simulink model "freq_detection_algorithm"  (R2021a)
settings: Solver=VariableStepAuto  StartTime=0.0  StopTime=10.0  RelTol=1e-3
Description:
  | Model is intend to simulate calculations for a flowmeter.
settings Model: Creator=Ayush  LastModifiedBy=Ayush

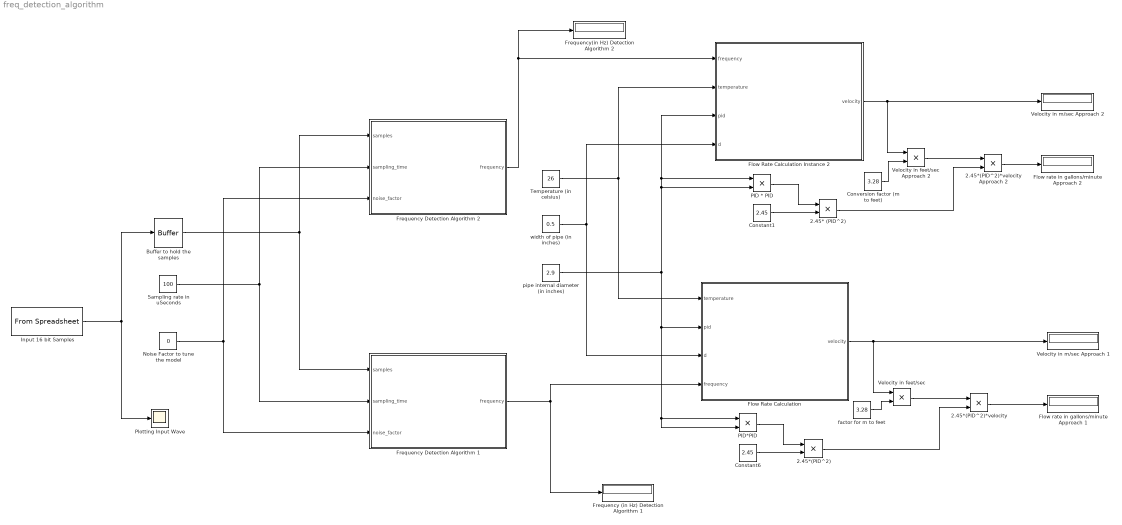
== system freq_detection_algorithm ==
  2.45* (PID^2) : Product
  2.45*(PID^2) : Product
  2.45*(PID^2)*velocity : Product
  2.45*(PID^2)*velocity Approach 2 : Product
  Buffer to hold the samples : Buffer  N=1000  OutputFrames=off
  Constant1 : Constant  Value=2.45  SampleTime=0.0005
  Constant6 : Constant  Value=2.45  SampleTime=0.0005
  Conversion factor (m to feet) : Constant  Value=3.28  SampleTime=0.0005
  Flow Rate Calculation : MATLAB Function  TreatAsAtomicUnit=on
  Flow Rate Calculation Instance 2 : MATLAB Function  TreatAsAtomicUnit=on
  Flow rate in gallons/minute Approach 1 : Display
  Flow rate in gallons/minute Approach 2 : Display
  Frequency (in Hz) Detection Algorithm 1 : Display
  Frequency Detection Algorithm 1 : MATLAB Function  TreatAsAtomicUnit=on
  Frequency Detection Algorithm 2 : MATLAB Function  TreatAsAtomicUnit=on
  Frequency(in Hz) Detection Algorithm 2 : Display
  Input 16 bit Samples : FromSpreadsheet  FileName=ECEN5803Data17_1.csv  SheetName=ECEN5803Data17_1  OutDataTypeStr=double  TreatFirstColumnAs=Data  SampleTime=0.0001
  Noise Factor to tune the model : Constant  Value=0  SampleTime=0.00001
  PID * PID : Product
  PID*PID : Product
  Plotting Input Wave : Scope
  Sampling rate in uSeconds : Constant  Value=100  SampleTime=100
  Temperature (in celsius) : Constant  Value=26  SampleTime=0.0005
  Velocity in feet/sec : Product
  Velocity in feet/sec Approach 2 : Product
  Velocity in m/sec Approach 1 : Display
  Velocity in m/sec Approach 2 : Display
  factor for m to feet : Constant  Value=3.28  SampleTime=0.0005
  pipe internal diameter (in inches) : Constant  Value=2.9  SampleTime=100
  width of pipe (in inches) : Constant  Value=0.5  SampleTime=100
  wires:
  Buffer to hold the samples/1 -> Frequency Detection Algorithm 2/1(samples), Frequency Detection Algorithm 1/1(samples)
  Sampling rate in uSeconds/1 -> Frequency Detection Algorithm 2/2(sampling_time), Frequency Detection Algorithm 1/2(sampling_time)
  Noise Factor to tune the model/1 -> Frequency Detection Algorithm 2/3(noise_factor), Frequency Detection Algorithm 1/3(noise_factor)
  Frequency Detection Algorithm 1/1(frequency) -> Flow Rate Calculation/4(frequency), Frequency (in Hz) Detection Algorithm 1/1
  Input 16 bit Samples/1 -> Buffer to hold the samples/1, Plotting Input Wave/1
  Flow Rate Calculation/1(velocity) -> Velocity in feet/sec/1, Velocity in m/sec Approach 1/1
  factor for m to feet/1 -> Velocity in feet/sec/2
  Velocity in feet/sec/1 -> 2.45*(PID^2)*velocity/1
  2.45*(PID^2)*velocity/1 -> Flow rate in gallons/minute Approach 1/1
  PID*PID/1 -> 2.45*(PID^2)/1
  Constant6/1 -> 2.45*(PID^2)/2
  2.45*(PID^2)/1 -> 2.45*(PID^2)*velocity/2
  Frequency Detection Algorithm 2/1(frequency) -> Frequency(in Hz) Detection Algorithm 2/1, Flow Rate Calculation Instance 2/1(frequency)
  2.45* (PID^2)/1 -> 2.45*(PID^2)*velocity Approach 2/2
  Constant1/1 -> 2.45* (PID^2)/2
  2.45*(PID^2)*velocity Approach 2/1 -> Flow rate in gallons/minute Approach 2/1
  Velocity in feet/sec Approach 2/1 -> 2.45*(PID^2)*velocity Approach 2/1
  Flow Rate Calculation Instance 2/1(velocity) -> Velocity in feet/sec Approach 2/1, Velocity in m/sec Approach 2/1
  PID * PID/1 -> 2.45* (PID^2)/1
  Temperature (in celsius)/1 -> Flow Rate Calculation/1(temperature), Flow Rate Calculation Instance 2/2(temperature)
  width of pipe (in inches)/1 -> Flow Rate Calculation Instance 2/4(d), Flow Rate Calculation/3(d)
  pipe internal diameter (in inches)/1 -> Flow Rate Calculation/2(pid), PID*PID/1, PID*PID/2, PID * PID/2, PID * PID/1, Flow Rate Calculation Instance 2/3(pid)
  Conversion factor (m to feet)/1 -> Velocity in feet/sec Approach 2/2

== matlab function freq_detection_algorithm/Frequency Detection Algorithm 1 ==
  data: samples input; frequency output; sampling_time input; noise_factor input
function frequency = frequency_detection3(samples, sampling_time, noise_factor)
    nsamples = length(samples);
    ntransitions = 0;
    nsamples_passed = 0;
    min_flag = 0;
    max_flag = 0;
    is_counting = 0;
    prev_sample_reading_taken = 0;
    for i = 2:nsamples
        if ((samples(i) - samples(i-1)) >= noise_factor)
            if (max_flag)
                max_flag = 0;
                if (is_counting)
                    ntransitions = ntransitions + 1;
                    nsamples_passed = nsamples_passed + i - prev_sample_reading_taken;
                    prev_sample_reading_taken = i;
                else
                    prev_sample_reading_taken = i;
                    is_counting = 1;
                end
            end
            min_flag = 1;
        elseif ((samples(i-1) - samples(i)) >= noise_factor)
            if (min_flag)
                min_flag = 0;
                if (is_counting)
                    ntransitions = ntransitions + 1;
                    nsamples_passed = nsamples_passed + i - prev_sample_reading_taken;
                    prev_sample_reading_taken = i;
                else
                    prev_sample_reading_taken = i;
                    is_counting = 1;
                end
            end
            max_flag = 1;
        end
    end
    if (ntransitions == 0) 
        frequency = 100;
    else
        frequency = (1000000/((nsamples_passed/ntransitions) * sampling_time * 2));

    end
    
end

== matlab function freq_detection_algorithm/Frequency Detection Algorithm 2 ==
  data: samples input; frequency output; sampling_time input; noise_factor input
function frequency = frequency_detection1(samples, sampling_time, noise_factor)
    nSamples = length(samples);
    total_time = 0;
    ncycles = 0;
    is_counting = 0;
    reference_value = samples(1);
    min_flag = 0;
    max_flag = 0;
    prev_sample_reading_taken = 0;
    nsamples_passed = 0;
    for i = 1:nSamples
        if (samples(i) - reference_value >= noise_factor)
            if (max_flag == 1)
                if is_counting== 1
                    ncycles = ncycles + 0.5;
                    nsamples_passed = nsamples_passed + i - prev_sample_reading_taken;
                    prev_sample_reading_taken = i;
                else
                    is_counting = 1;
                    prev_sample_reading_taken = i;
                    reference_value = samples(i);
                end
                max_flag = 0;                
            end
            min_flag = 1;
        elseif (reference_value - samples(i) > noise_factor)
            if (min_flag == 1)
                if is_counting== 1
                    ncycles = ncycles + 0.5;
                    nsamples_passed = nsamples_passed + i - prev_sample_reading_taken;
                    prev_sample_reading_taken = i;
                else
                    is_counting = 1;
                    prev_sample_reading_taken = i;
                    reference_value = samples(i);
                end
                min_flag = 0;
            end
            max_flag = 1;
        end
    end
    if ncycles
        frequency = (1000000/((nsamples_passed/ncycles) * sampling_time));
    else
        frequency = 100;
    end
end

== matlab function freq_detection_algorithm/Flow Rate Calculation ==
  data: temperature input; pid input; d input; frequency input; velocity output
function velocity = flow_rate_calculation(temperature, pid, d, frequency)
    %velocity is in m/sec
    %frequency in Hz
    %temperature in celsius
    %
    pid = pid * 0.0254; % convert to meters
    d = d * 0.0254; %converts to meters
    T = temperature + 273.15; % converts the temperature to Kelvin
    density = 1000*(1 - ((temperature + 288.9414)/(508929.2* (temperature + 68.1293))) * ((temperature-3.9862)^2));
    viscosity = (2.4 * 10^(-5)) * (10 ^((247.8/(T - 140))));
    
    a = 0.0671;
    b = -1*((0.05368*frequency*d) + (viscosity / (density*pid)));
    c = (frequency*d)^2;
    
    p = [a b c];
    r = roots(p);
    absolute_values = abs(r);
    v = absolute_values(1)
    
    velocity = v;
end

== matlab function freq_detection_algorithm/Flow Rate Calculation Instance 2 ==
  data: frequency input; temperature input; pid input; d input; velocity output
function velocity = flow_rate_calculation(frequency, temperature, pid, d)
    %velocity is in m/sec
    %frequency in Hz
    %temperature in celsius
    %
    pid = pid * 0.0254; % convert to meters
    d = d * 0.0254; %converts to meters
    T = temperature + 273.15; % converts the temperature to Kelvin
    density = 1000*(1 - ((temperature + 288.9414)/(508929.2* (temperature + 68.1293))) * ((temperature-3.9862)^2));
    viscosity = (2.4 * 10^(-5)) * (10 ^((247.8/(T - 140))));
    
    a = 0.0671;
    b = -1*((0.05368*frequency*d) + (viscosity / (density*pid)));
    c = (frequency*d)^2;
    
    p = [a b c];
    r = roots(p);
    absolute_values = abs(r);
    v = absolute_values(1)
    
    velocity = v;
end
